simulink model "allModel_V1slx"  (R2023b)
settings: Solver=FixedStepAuto  StartTime=0.0  StopTime=data.tVec(end)  FixedStep=Ts_sim  RelTol=1e-3
values from neighbouring files (symbols this model uses):
  T_amb = 23    [Sim_bothLoop_compare.m]    (also in ident_All_V6.m; reportScript.m)
undefined symbols (not defined in the file or in its folder): sysTMC
libraries: cstblocks x2
settings Model: Creator=maxja  LastModifiedBy=maxja

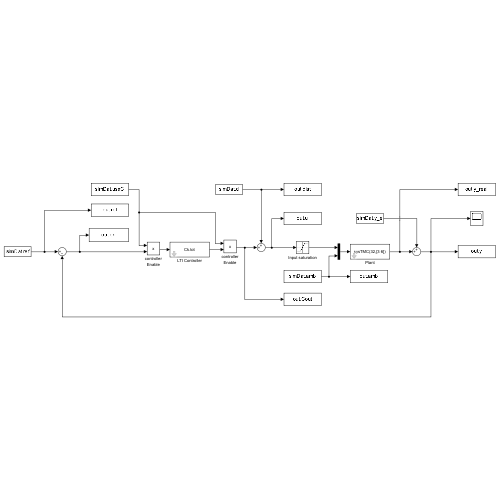
[thumbnail: Simulink's stored preview of the top-level diagram]
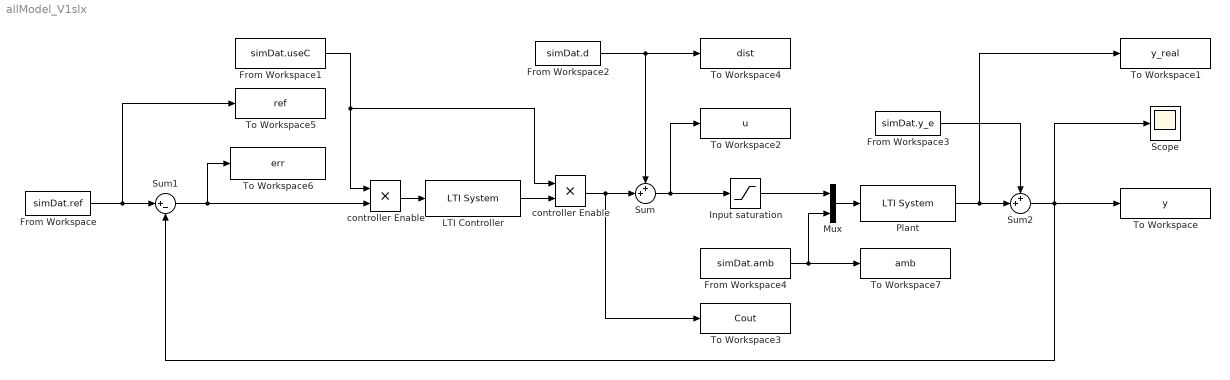
== system allModel_V1slx ==
  From Workspace : FromWorkspace  VariableName=simDat.ref
  From Workspace1 : FromWorkspace  VariableName=simDat.useC
  From Workspace2 : FromWorkspace  VariableName=simDat.d
  From Workspace3 : FromWorkspace  VariableName=simDat.y_e
  From Workspace4 : FromWorkspace  VariableName=simDat.amb
  Input saturation : Saturate  UpperLimit=inf  LowerLimit=0
  LTI Controller : cstblocks/LTI System  sys=Ck.tot  IC=[]  PadeOrder=0
  Mux : Mux  Inputs=2
  Plant : cstblocks/LTI System  sys=sysTMC(32,[3 6])  IC=[T_amb.*ones(218,1)]  PadeOrder=0
  Scope : Scope
  Sum : Sum  Inputs=++|
  Sum1 : Sum  Inputs=|+-
  Sum2 : Sum  Inputs=++|
  To Workspace : ToWorkspace  VariableName=y  SaveFormat=Timeseries  SampleTime=-1
  To Workspace1 : ToWorkspace  VariableName=y_real  SaveFormat=Timeseries  SampleTime=-1
  To Workspace2 : ToWorkspace  VariableName=u  SaveFormat=Timeseries  SampleTime=-1
  To Workspace3 : ToWorkspace  VariableName=Cout  SaveFormat=Timeseries  SampleTime=-1
  To Workspace4 : ToWorkspace  VariableName=dist  SaveFormat=Timeseries  SampleTime=-1
  To Workspace5 : ToWorkspace  VariableName=ref  SaveFormat=Timeseries  SampleTime=-1
  To Workspace6 : ToWorkspace  VariableName=err  SaveFormat=Timeseries  SampleTime=-1
  To Workspace7 : ToWorkspace  VariableName=amb  SaveFormat=Timeseries  SampleTime=-1
  controller Enable : Product
  "controller Enable " : Product
  wires:
  From Workspace/1 -> To Workspace5/1, Sum1/1
  LTI Controller/1 -> controller Enable/2
  controller Enable/1 -> To Workspace3/1, Sum/2
  Sum/1 -> Input saturation/1, To Workspace2/1
  From Workspace1/1 -> "controller Enable "/1, controller Enable/1
  From Workspace2/1 -> To Workspace4/1, Sum/1
  Sum1/1 -> "controller Enable "/2, To Workspace6/1
  Plant/1 -> To Workspace1/1, Sum2/2
  From Workspace3/1 -> Sum2/1
  Sum2/1 -> Sum1/2, Scope/1, To Workspace/1
  "controller Enable "/1 -> LTI Controller/1
  Input saturation/1 -> Mux/1
  From Workspace4/1 -> To Workspace7/1, Mux/2
  Mux/1 -> Plant/1
